simulink model "Main"  (R2020b)
settings: Solver=FixedStepAuto  StartTime=0.0  StopTime=80  FixedStep=0.001  RelTol=1e-3
model workspace (MAT data in the model file):
  fd = 1
settings Model: Creator=kaebi  LastModifiedBy=kaebi
settings ConfigComp: PLC_TargetIDE=twincat3

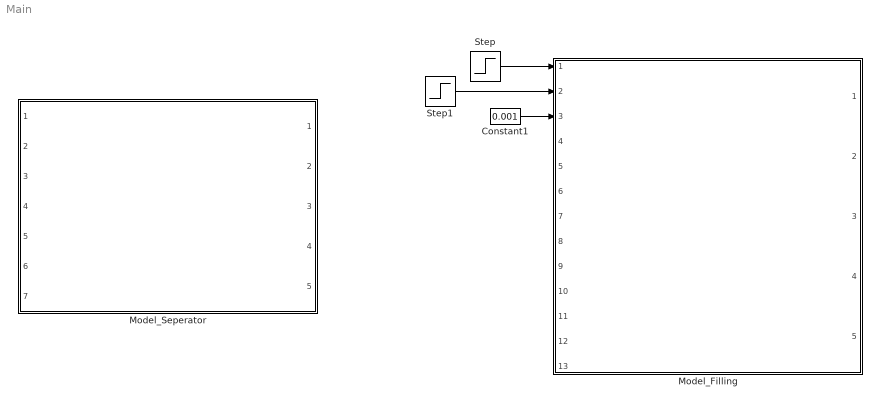
== system Main ==
  Constant1 : Constant  Value=0.001
  Model_Filling : Subsystem  TreatAsAtomicUnit=on  ReferencedSubsystem=SubSystemBefullung
  Model_Seperator : Subsystem  TreatAsAtomicUnit=on  ReferencedSubsystem=SubSystemVereinzelung
  Step : Step  Time=0.01  SampleTime=0
  Step1 : Step  Time=0.015  SampleTime=0
  wires:
  Constant1/1 -> Model_Filling/3
  Step/1 -> Model_Filling/1
  Step1/1 -> Model_Filling/2
